simulink model "eml_clock"  (R2015a)
settings: Solver=ode45  StartTime=0.0  StopTime=inf  RelTol=1e-3
StopFcn:
  | obj = findobj( 'Tag', 'emlclock_fig');
  | if ~isempty(obj),
  |    close(obj);
  | end;
settings Model: CovSFcnEnable=off  ExtModeAutoUpdateStatusClock=off  Creator=The MathWorks, Inc.  LastModifiedBy=ktrinh
settings DataIOCC: SignalLoggingName=logsOut
settings OptimizationCC: ExpressionDepthLimit=2147483647  InitFltsAndDblsToZero=on
settings DebuggingCC: UnderspecifiedInitializationDetection=Classic  MergeDetectMultiDrivingBlocksExec=none  CheckExecutionContextPreStartOutputMsg=on  CheckExecutionContextRuntimeOutputMsg=on  SignalResolutionControl=TryResolveAllWithWarning  MultiTaskDSMMsg=warning  MultiTaskCondExecSysMsg=none  FcnCallInpInsideContextMsg=EnableAllAsWarning  StateNameClashWarn=warning
settings ModelReferenceCC: UpdateModelReferenceTargets=IfOutOfDate
settings SFSimCC: SimParseCustomCode=off
settings GRTTargetCC: CombineOutputUpdateFcns=off  GRTInterface=on

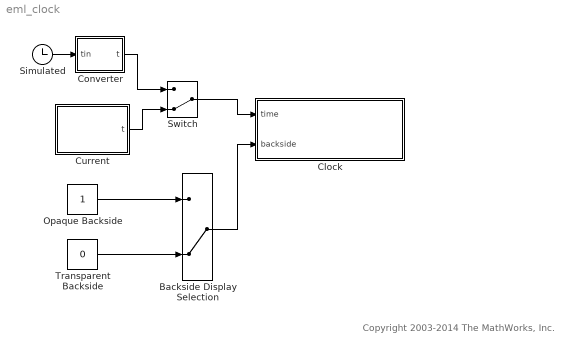
== system eml_clock ==
  note: Copyright 2003-2014 The MathWorks, Inc.
  Backside Display Selection : ManualSwitch  CurrentSetting=0
  Clock : MATLAB Function  TreatAsAtomicUnit=on
      settings: PermitHierarchicalResolution=ParametersOnly
  Converter : MATLAB Function  TreatAsAtomicUnit=on
      settings: PermitHierarchicalResolution=ParametersOnly
  Current : MATLAB Function  TreatAsAtomicUnit=on
      settings: PermitHierarchicalResolution=ParametersOnly
  Opaque Backside : Constant  OutDataTypeStr=double
  Simulated : Clock
  Switch : ManualSwitch  CurrentSetting=0
  Transparent Backside : Constant  Value=0  OutDataTypeStr=double
  wires:
  Switch/1 -> Clock/1(time)
  Current/1(t) -> Switch/2
  Converter/1(t) -> Switch/1
  Simulated/1 -> Converter/1(tin)
  Opaque Backside/1 -> Backside Display Selection/1
  Transparent Backside/1 -> Backside Display Selection/2
  Backside Display Selection/1 -> Clock/2(backside)

== matlab function eml_clock/Current ==
  data: t output double
function t = time
coder.extrinsic('clock','fix');
t = [0,0,0,0,0,0];
t = fix(clock);
t(4) = t(4) + t(5)/60;

== matlab function eml_clock/Clock ==
  settings: updateMethod=DISCRETE
  data: time input double; backside input double
function emlclock(time,backside)
persistent initialized;
persistent fig;
persistent fig_axes;
persistent bag_board_front;
persistent bag_board_back;
persistent bag_hands;
persistent hour_hand_id;
persistent minute_hand_id;
persistent second_hand_id;
persistent front_visible;
persistent iteration;
persistent old_backside;
persistent old_front_visible;

coder.extrinsic('figure','set','hold','patch','plot3');

%assert(isa(time, 'double'));
%assert(all(size(time) == [1 6]));
%assert(isa(backside, 'double'));

if isempty(initialized)
    initialized = 1;
    iteration = 0;
    old_front_visible = 0;
    old_backside = backside;
    
    fig = figure;
    set(fig, 'DoubleBuffer', 'on', 'Tag', 'emlclock_fig');
    hold('on');
    fig_axes = get(fig, 'CurrentAxes');
    init_axes( fig_axes );
    
    bag_board_front = create_empty_bag;
    bag_board_front = append_bag( bag_board_front, create_analogue_board );

    bag_board_back = create_empty_bag;
    bag_board_back = create_board_background( bag_board_back );
    
    bag_hands = create_empty_bag;
    hour_hand_id = next_bag_id(bag_hands);
    bag_hands = create_hour_hand(bag_hands);
    minute_hand_id = next_bag_id(bag_hands);
    bag_hands = create_minute_hand(bag_hands);
    second_hand_id = next_bag_id(bag_hands);
    bag_hands = create_second_hand(bag_hands);
    
    update_bag(bag_board_front);
    update_bag(bag_board_back);
    update_bag(bag_hands);
else
    full_update = 0;
    if old_backside ~= backside,
        full_update = 1;
        old_backside = backside;
    end;
    
    t = [0,0,0,0,0,0];
    t = time;

    bag_hands = set_item_argument( bag_hands, hour_hand_id, -t(4)*2*pi/12 );
    bag_hands = set_item_argument( bag_hands, minute_hand_id, -t(5)*2*pi/60 );
    bag_hands = set_item_argument( bag_hands, second_hand_id, -t(6)*2*pi/60 );
    
    camera_argument = rem(2*pi*iteration / 200, 2*pi);
    camera_position = 200*[cos(camera_argument),0,sin(camera_argument)];
    set(fig_axes, 'CameraPosition', camera_position);

    if camera_argument < pi,
        front_visible = 1;
    else
        front_visible = 0;
    end;
    
    if ~backside,
        front_visible = 1;
    end;
    
    if front_visible ~= old_front_visible,
        old_front_visible = front_visible;
        full_update = 1;
    end;
    
    if full_update,
        bag_hands = set_bag_visibility( bag_hands, front_visible );
        bag_board_front = set_bag_visibility( bag_board_front, front_visible );
        bag_board_back = set_bag_visibility( bag_board_back, double(~front_visible) );
        update_bag( bag_hands );
        update_bag( bag_board_front );
        update_bag( bag_board_back );
    else
        update_bag( bag_hands );
    end;
    
    iteration = iteration + 1;
end;

function init_axes(a)
    coder.extrinsic('set');
    set(a, 'CameraTarget', [0,0,0] );
    set(a, 'CameraPosition', [0,0,300]);
    set(a, 'CameraViewAngle', 80 );
    set(a, 'CameraUpVector', [0,1,0]);
    set(a, 'Visible', 'off' ); 
    set(a, 'ALimMode', 'manual' );
    set(a, 'XLimMode', 'manual');
    set(a, 'YLimMode', 'manual');
    set(a, 'XLim', [-150,150]);
    set(a, 'YLim', [-150,150]);
    set(a, 'ZLim', [-150,150]);

function r = create_empty_patch
    coder.extrinsic('patch');
    r = patch([0],[0],[0],[0,0,0]);

function r = create_empty_plot
    coder.extrinsic('plot3');
    r = plot3([0],[0],[0]);    
    
function bag = create_empty_bag 
    coder.extrinsic('feval');
    n = 400;
    bag = feval('cell', 1, n);
    bag = set_bag_element(bag, 1, 1);
    for i = 2:n
        bag = set_bag_element(bag, i, 0);
    end

function bag = set_bag_element(bag, index, value)    
    coder.extrinsic('subsasgn', 'num2cell');
    bag = subsasgn(bag, struct('type', '{}', 'subs', num2cell(num2cell(index))), value);

function value = get_bag_element(bag, index)
    coder.extrinsic('subsref', 'num2cell');
    value = subsref(bag, struct('type', '{}', 'subs', num2cell(num2cell(index))));
    
function r = bag_size(bag)
    coder.extrinsic('subsref', 'num2cell');
    r = 0;
    r = get_bag_element(bag, 1);
    
function r = next_bag_id(bag)
    r = bag_size(bag) + 1;

function bag = update_bag_size(bag,siz)
    coder.extrinsic('subsasgn', 'num2cell');
    bag = subsasgn(bag, struct('type', '{}', 'subs', num2cell(num2cell(1))), siz);
    
function update_bag(bag)    
    p = 2;
    p_end = bag_size(bag);
    while p <= p_end,
        update_item_d(bag, p, 0, [0,0,0]);
        itemSize = 0;
        itemSize = get_bag_element(bag,p+1);
        p = p + itemSize + item_base_size;
    end;
    
function update_item(bag,id)
    update_item_d(bag,id,0,[0,0,0]);
    
function update_item_d(bag,id,arg,offset)
    type = 0;
    type = get_bag_element(bag,id);
    switch type
        case 0
            update_inner_bag(bag,id,arg,offset);
        otherwise
            update_item_d1(bag,id,arg,offset);
            arg0 = 0;
            arg0 = get_bag_element(bag,id+2);
            rotate_item(bag,id,arg+arg0,offset);
            update_item_visibility(bag,id);
    end;

function update_item_d1(bag,id,arg,offset)
    type = 0;
    type = get_bag_element(bag, id);
    switch type
        case 1
            update_hour_hand(bag,id,offset);
        case 2
            update_minute_hand(bag,id,offset);
        case 3
            update_second_hand(bag,id,offset);
        case 4
            update_x_glyph(bag,id,offset);
        case 5
            update_v_glyph(bag,id,offset);
        case 6
            update_i_glyph(bag,id,offset);
        case 7
            update_board_background(bag,id,offset);
    end;
    
function r = update_inner_bag(bag,id,arg,offset)
    siz = 0;
    siz = get_bag_element(bag,id+1);
    newarg = 0;
    newarg = get_bag_element(bag,id+2);
    newarg = newarg + arg;
    x = 0;
    x = get_bag_element(bag,id+3);
    x = x + offset(1);
    y = 0;
    y = get_bag_element(bag,id+4);
    y = y + offset(2);
    z = 0;
    z = get_bag_element(bag,id+5);
    z = z + offset(3);
    p = item_base_size + id;
    p_end = p + siz;
    while p < p_end,
        update_item_d1(bag, p, newarg, [x,y,z]);
        p1 = 0;
        p1 = get_bag_element(bag,p+1);
        p = p + p1 + item_base_size;
    end;

function rotate_item(bag,id,arg,offset)
    coder.extrinsic('rotate');
    item_size = 0;
    item_size = get_bag_element(bag,id+1);
    p = id + item_base_size;
    p_end = p + item_size;
    while p < p_end,
        bagp = get_bag_element(bag,p);
        rotate( bagp, [0,0,1], 360*arg/2/pi );
        p = p + 1;
    end;

function update_item_visibility(bag,id)
    coder.extrinsic('set');
    item_size = 0;
    item_size = get_bag_element(bag,id+1);
    visibility = 0;
    visibility = get_bag_element(bag,id+6);
    p = id + item_base_size;
    p_end = p + item_size;
    if visibility == 1,
        while p < p_end,
            h = get_bag_element(bag,p);
            set( h, 'Visible', 'on' );
            p = p + 1;
        end;
    else
        while p < p_end,
            h = get_bag_element(bag,p);
            set( h, 'Visible', 'off' );
            p = p + 1;
        end;
    end;

function bag = add_item(bag,type,size)
    coder.extrinsic('subsasgn', 'num2cell');
    id = next_bag_id(bag);
    bag = subsasgn(bag, struct('type', '{}', 'subs', num2cell(num2cell(id))), type);
    bag = subsasgn(bag, struct('type', '{}', 'subs', num2cell(num2cell(id+1))), size);
    for i = 2:5
        % Argument, X Position, Y Position, Z Position = 0
        bag = subsasgn(bag, struct('type', '{}', 'subs', num2cell(num2cell(id+i))), 0);
    end
    bag = update_bag_size(bag, bag_size(bag) + item_base_size + size);
    
function r = item_base_size
    r = 7;
    
function bag = copy_item(bag, bag_source, p)
    siz = bag_size(bag);
    for i = 1:item_base_size,
        bag = set_bag_element(bag, siz+i, get_bag_element(bag_source,p+i-1));
    end;
    siz = siz + item_base_size;
    item_siz = 0;
    item_siz = get_bag_element(bag_source,p+1);
    p = p + item_base_size;
    for i = 1:item_siz,
        bag = set_bag_element(bag,siz+i,get_bag_element(bag_source,p+i-1));
    end;
    bag = update_bag_size(bag, item_siz + siz);

function bag = set_item_argument(bag,id,arg)
    bag = set_bag_element(bag,id+2,arg);
        
function bag = set_item_position(bag,id,pos)
    bag = set_bag_element(bag,id+3,pos(1));
    bag = set_bag_element(bag,id+4,pos(2));
    bag = set_bag_element(bag,id+5,pos(3));

function bag = set_item_visibility(bag,id,visible)
    bag = set_bag_element(bag,id+6,visible);
    
function bag = create_hour_hand(bag)
    id = next_bag_id(bag);
    bag = add_item(bag,1,1);
    i = id + item_base_size;
    bag = set_bag_element(bag,i,create_empty_patch);
    
function update_hour_hand(bag,id,offset)
    coder.extrinsic('set');
    i = id + item_base_size;
    x = 0;
    x = get_bag_element(bag, id+3);
    x = x + offset(1);
    y = 0;
    y = get_bag_element(bag, id+4);
    y = y + offset(2);
    z = 0;
    z = get_bag_element(bag, id+5);
    z = z + offset(3);
    h = get_bag_element(bag, i);
    set(h, 'XData', [0,-10,0,10,0] + x);
    set(h, 'YData', [0,70,80,70,0] + y);
    set(h, 'ZData', [0,0,0,0,0] + z);
    set(h, 'FaceColor', [1.0,0,0] );    
    
function bag = create_minute_hand(bag)
    id = next_bag_id(bag);
    bag = add_item(bag,2,1);
    i = id + item_base_size;
    bag = set_bag_element(bag,i,create_empty_patch);

function update_minute_hand(bag,id,offset)
    coder.extrinsic('set');
    i = id + item_base_size;
    x = 0;
    x = get_bag_element(bag, id+3);
    x = x + offset(1);
    y = 0;
    y = get_bag_element(bag, id+4);
    y = y + offset(2);
    z = 0;
    z = get_bag_element(bag, id+5);
    z = z + offset(3);
    h = get_bag_element(bag, i);
    set(h, 'XData', [0,-10,0,10,0] + x);
    set(h, 'YData', [0,100,110,100,0] + y);
    set(h, 'ZData', [0,0,0,0,0] + z);
    set(h, 'FaceColor', [1.0,0,0] );

function bag = create_second_hand(bag)
    id = next_bag_id(bag);
    bag = add_item(bag,3,1);
    i = id + item_base_size;
    bag = set_bag_element(bag,i,create_empty_patch);
    
function update_second_hand(bag,id,offset)
    coder.extrinsic('set');
    i = id + item_base_size;
    x = 0;
    x = get_bag_element(bag, id+3);
    x = x + offset(1);
    y = 0;
    y = get_bag_element(bag, id+4);
    y = y + offset(2);
    z = 0;
    z = get_bag_element(bag, id+5);
    z = z + offset(3);
    h = get_bag_element(bag, i);
    set(h, 'XData', [0,-3,0,3,0]+x );
    set(h, 'YData', [0,100,110,100,0]+y );
    set(h, 'ZData', [0,0,0,0,0]+z );
    set(h, 'FaceColor', [0,1.0,0] );

function r = get_roman(n)
    switch (n)
        case 1
            r = 'I   ';
        case 2
            r = 'II  ';
        case 3
            r = 'III ';
        case 4
            r = 'IV  ';
        case 5
            r = 'V   ';
        case 6
            r = 'VI  ';
        case 7
            r = 'VII ';
        case 8
            r = 'VIII';
        case 9
            r = 'XI  ';
        case 10
            r = 'X   ';
        case 11
            r = 'XI  ';
        case 12
            r = 'XII ';
        otherwise
            r = '    ';
    end;
    
function r = create_analogue_board
    bag = create_empty_bag;
    for i = 1:12,
        str = get_roman(i);
        bag0 = create_string(str);
        pos = 95*[cos(-(i-3)*2*pi/12),sin(-(i-3)*2*pi/12),0];
        bag0 = move_bag( bag0, pos );
        bag = append_bag(bag,bag0);
    end;
    bag = create_board_background(bag);
    r = bag;
    
function r = create_string(str)
    bag = create_empty_bag;
    pos_x = 0;
    for c = str,
        ok = 0;
        id = next_bag_id(bag);
        switch c
            case 'X'
                bag = create_x_glyph(bag);
                ok = 1;
            case 'V'
                bag = create_v_glyph(bag);
                ok = 1;
            case 'I'
                bag = create_i_glyph(bag);
                ok = 1;
        end;
        if ok,
            bag = set_item_position(bag,id,[pos_x,0.3*-30,0]);
            step = 0.3*55;
            if c == 'I',
                step = 0.3*20;
            end;
            pos_x = pos_x + step;
        end;
    end;
    bag = move_bag( bag, [-pos_x/2,0,0] );
    r = bag;

function r = append_bag(bag,bag0)
    id = next_bag_id(bag);
    siz0 = bag_size(bag0);
    p = 2;
    while p < siz0,
        bag = copy_item( bag, bag0, p );
        item_size = 0;
        item_size = get_bag_element(bag0,p+1);
        p = p + item_size + item_base_size;
    end;
    r = bag;
    
function bag = move_bag(bag,delta)
    dx = delta(1);
    dy = delta(2);
    dz = delta(3);
    siz = bag_size(bag);
    p = 2;
    p_end = p + siz;
    while p < p_end,
        item_size = 0;
        item_size = get_bag_element(bag,p+1);
        x = 0;
        y = 0;
        z = 0;
        x = get_bag_element(bag,p+3);
        y = get_bag_element(bag,p+4);
        z = get_bag_element(bag,p+5);
        bag = set_bag_element(bag, p+3, x+dx);
        bag = set_bag_element(bag, p+4, y+dy);
        bag = set_bag_element(bag, p+5, z+dz);
        p = p + item_size + item_base_size;
    end;

function r = set_bag_visibility(bag,visible)
    siz = bag_size(bag);
    p = 2;
    p_end = p + siz;
    while p < siz,
        item_size = 0;
        item_size = get_bag_element(bag,p+1);
        bag = set_bag_element(bag,p+6,visible);
        p = p + item_size + item_base_size;
    end;
    r = bag;
    
function print_bag(bag)
    coder.extrinsic('fprintf');
    siz = bag_size(bag);
    p = 2;
    while p < siz,
        item_type = bag(p);
        item_size = bag(p+1);
        item_arg = bag(p+2);
        item_x = bag(p+3);
        item_y = bag(p+4);
        item_z = bag(p+5);
        fprintf( 1, 'type=%d, arg=%d, pos=[%d,%d,%d]\n',...
                    item_type, item_arg, item_x, item_y, item_z );
        p = p + item_size + item_base_size;
    end;
    
function bag = create_x_glyph(bag)
    id = next_bag_id(bag);
    bag = add_item(bag,4,1);
    i = id + item_base_size;
    bag = set_bag_element(bag, i, create_empty_patch);

function update_x_glyph(bag,id,offset)
    coder.extrinsic('set');
    i = id + item_base_size;
    x = 0;
    x = get_bag_element(bag,id+3);
    x = x + offset(1);
    y = 0;
    y = get_bag_element(bag,id+4);
    y = y + offset(2);
    z = 0;
    z = get_bag_element(bag,id+5);
    z = z + offset(3);
    h = get_bag_element(bag, i);
    set(h, 'XData', 0.3*[0,20,0,10,25,40,50,30,50,40,25,10,0]+x );
    set(h, 'YData', 0.3*[0,30,60,60,40,60,60,30,0,0,20,0,0]+y );
    set(h, 'ZData', 0.3*[0,0,0,0,0,0,0,0,0,0,0,0,0]+z );
    set(h, 'FaceColor', [0,0,1.0] );

function bag = create_v_glyph(bag)
    id = next_bag_id(bag);
    bag = add_item(bag,5,1);
    i = id + item_base_size;
    bag = set_bag_element(bag, i, create_empty_patch);

function update_v_glyph(bag,id,offset)
    coder.extrinsic('set');
    i = id + item_base_size;
    x = 0;
    x = get_bag_element(bag,id+3);
    x = x + offset(1);
    y = 0;
    y = get_bag_element(bag,id+4);
    y = y + offset(2);
    z = 0;
    z = get_bag_element(bag,id+5);
    z = z + offset(3);
    h = get_bag_element(bag, i);
    set(h, 'XData', 0.3*[0,10,25,40,50,25,0]+x );
    set(h, 'YData', 0.3*[60,60,20,60,60,0,60]+y );
    set(h, 'ZData', 0.3*[0,0,0,0,0,0,0]+z );
    set(h, 'FaceColor', [0,0,1.0] );

function bag = create_i_glyph(bag)
    id = next_bag_id(bag);
    bag = add_item(bag,6,1);
    i = id + item_base_size;
    bag = set_bag_element(bag, i, create_empty_patch);
    
function update_i_glyph(bag,id,offset)
    coder.extrinsic('set');
    i = id + item_base_size;
    x = 0;
    x = get_bag_element(bag,id+3);
    x = x + offset(1);
    y = 0;
    y = get_bag_element(bag,id+4);
    y = y + offset(2);
    z = 0;
    z = get_bag_element(bag,id+5);
    z = z + offset(3);
    h = get_bag_element(bag, i);
    set(h, 'XData', 0.3*[0,10,10,0,0]+x );
    set(h, 'YData', 0.3*[60,60,0,0,60]+y );
    set(h, 'ZData', 0.3*[0,0,0,0,0]+z );
    set(h, 'FaceColor', [0,0,1.0] );

function bag = create_board_background(bag)
    id = next_bag_id(bag);
    bag = add_item(bag,7,1);
    i = id + item_base_size;
    bag = set_bag_element(bag,i,create_empty_plot);
    
function r = update_board_background(bag,id,offset)
    coder.extrinsic('set');
    i = id + item_base_size;
    x = 0;
    x = get_bag_element(bag,id+3);
    x = x + offset(1);
    y = 0;
    y = get_bag_element(bag,id+4);
    y = y + offset(2);
    z = 0;
    z = get_bag_element(bag,id+5);
    z = z + offset(3);
    r = 0:pi/50:2*pi+pi/50;
    xdata = 110*cos(r);
    ydata = 110*sin(r);
    zdata = 0*r;
    h = get_bag_element(bag,i);
    set(h, 'XData', xdata+x );
    set(h, 'YData', ydata+y );
    set(h, 'ZData', zdata+z );
    set(h, 'Color', [0,0,1.0] );

== matlab function eml_clock/Converter ==
  data: tin input double; t output double
function t = conv(tin)
xhrs = rem(tin / 3600,24);
xmin = rem(tin / 60,60);
xsec = rem(tin,60);
t = [0,0,0,xhrs,xmin,xsec];
